simulink model "mcb_hostmodel_dsPIC33A"  (R2025b)
settings: Solver=FixedStepDiscrete  StartTime=0.0  StopTime=inf  RelTol=1e-3  EnableMultiTasking=on
values from neighbouring files (symbols this model uses):
  Ts_serialOut = 500e-6    (= 0.0005)    [mchp_acim_foc_dsPIC33A_data.m]
undefined symbols (not defined in the file or in its folder): target
libraries: instrumentseriallib x3, simulink x3
settings Model: Creator=The MathWorks, Inc.  LastModifiedBy=I73849
settings SolverCC: AlgebraicLoopSolver=TrustRegion  MaxZcPerStep=1.0
settings DataIOCC: LimitDataPoints=on  SaveFormat=Array  ReturnWorkspaceOutputs=off
settings OptimizationCC: ReuseModelBlockBuffer=off  LifeSpan=1  EfficientTunableParamExpr=on
settings DebuggingCC: UnderspecifiedInitializationDetection=Classic  MergeDetectMultiDrivingBlocksExec=none  SolverPrmCheckMsg=warning  ParameterPrecisionLossMsg=none  UnconnectedInputMsg=warning  UnconnectedOutputMsg=warning  UnconnectedLineMsg=warning  AllowSymbolicDim=off  PregeneratedLibrarySubsystemCodeDiagnostic=none  SFUnexpectedBacktrackingDiag=warning  SFNoUnconditionalDefaultTransitionDiag=warning  SFExecutionAtInitializationDiag=none  ArithmeticOperatorsInVariantConditions=warning
settings HardwareCC: ProdBitPerPointer=32.0  ProdLargestAtomicFloat=None  ProdIntDivRoundTo=Undefined  ProdEndianess=Unspecified  ProdWordSize=32.0  ProdHWDeviceType=32-bit Generic
settings ModelReferenceCC: EnableRefExpFcnMdlSchedulingChecks=on  PropagateSignalLabelsOutOfModel=off
settings SFSimCC: SimUseLocalCustomCode=off  MATLABDynamicMemAlloc=off
settings RTWCC: SystemTargetFile=ert.tlc  TemplateMakefile=ert_default_tmf  GenerateReport=on  RTWUseLocalCustomCode=off  IncludeHyperlinkInReport=on  LaunchReport=on  GenerateTraceInfo=on  GenerateTraceReport=on  GenerateTraceReportSl=on  GenerateTraceReportSf=on  GenerateTraceReportEml=on  GPUComputeCapability=3.5  DLArmComputeVersion=19.05  Description=Real-Time Workshop Embedded Coder
settings CodeAppCC: IgnoreCustomStorageClasses=off  StateflowObjectComments=on  InternalIdentifier=Classic
settings ERTTargetCC: InlinedParameterPlacement=Hierarchical  ERTCustomFileTemplate=example_file_process.tlc  ConvertIfToSwitch=off  SuppressUnreachableDefaultCases=off  DynamicArrayContainerType=coder::array  MultiwordLength=2048.0  GenerateSampleERTMain=on
settings ConfigComp: CovMetricSettings=dw  CovSaveCumulativeToWorkspaceVar=on  CovSaveSingleToWorkspaceVar=on  CovExternalEMLEnable=off  CovSFcnEnable=off

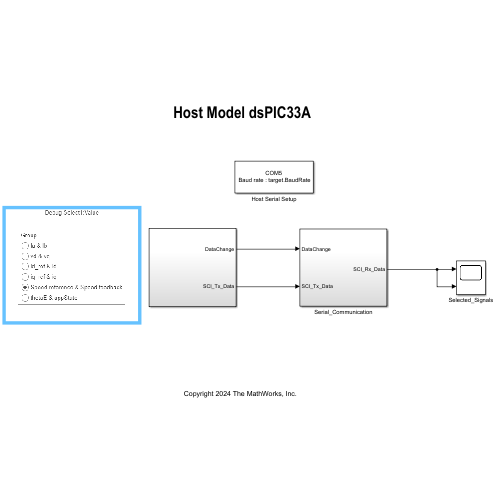
[thumbnail: Simulink's stored preview of the top-level diagram]
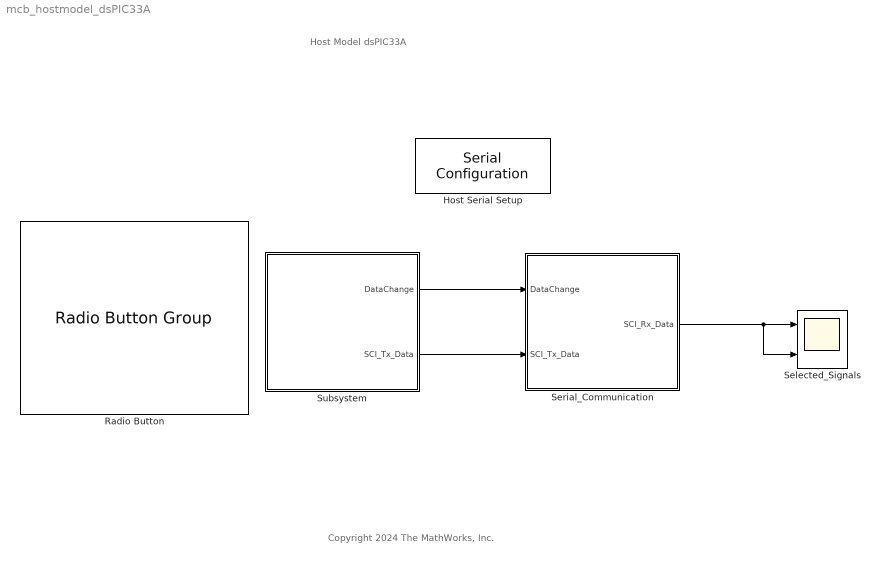
== system mcb_hostmodel_dsPIC33A ==
  note: Host Model dsPIC33A
  note: Copyright 2024 The MathWorks, Inc.
  Host Serial Setup : instrumentseriallib/Serial Configuration  Priority=-99  PortSel=target.comport  Port=target.comport  ComPort=target.comport  BaudRate=target.BaudRate  DataBits=8  Parity=none  StopBits=1  ByteOrder=little-endian  FlowControl=none  Timeout=2  SimulateUsing=Interpreted execution  BlockInModel=on  aMode=5
  Radio Button : RadioButtonGroup  SelectedLabel=Speed reference & Speed feedback  ButtonGroupName=Group
  Selected_Signals : Scope  NumInputPorts=2
      settings: TimeSpan=4  ActiveDisplayYMinimum=-510.99130861461151  ActiveDisplayYMaximum=4605.8121853321791  DataLoggingVariableName=Results_HW
  Serial_Communication : Subsystem
  Subsystem : Subsystem
  wires:
  Subsystem/2(SCI_Tx_Data) -> Serial_Communication/2(SCI_Tx_Data)
  Subsystem/1(DataChange) -> Serial_Communication/1(DataChange)
  Serial_Communication/1(SCI_Rx_Data) -> Selected_Signals/2, Selected_Signals/1

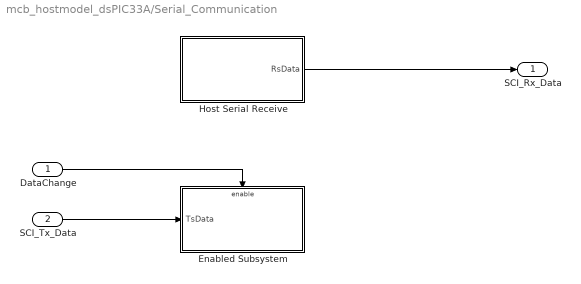
== system mcb_hostmodel_dsPIC33A/Serial_Communication ==
  DataChange : Inport
  SCI_Tx_Data : Inport  Port=2
  Enabled Subsystem : Subsystem  TreatAsAtomicUnit=on
  Host Serial Receive : Subsystem
  SCI_Rx_Data : Outport
  wires:
  DataChange/1 -> Enabled Subsystem/Enable
  SCI_Tx_Data/1 -> Enabled Subsystem/1(TsData)
  Host Serial Receive/1(RsData) -> SCI_Rx_Data/1

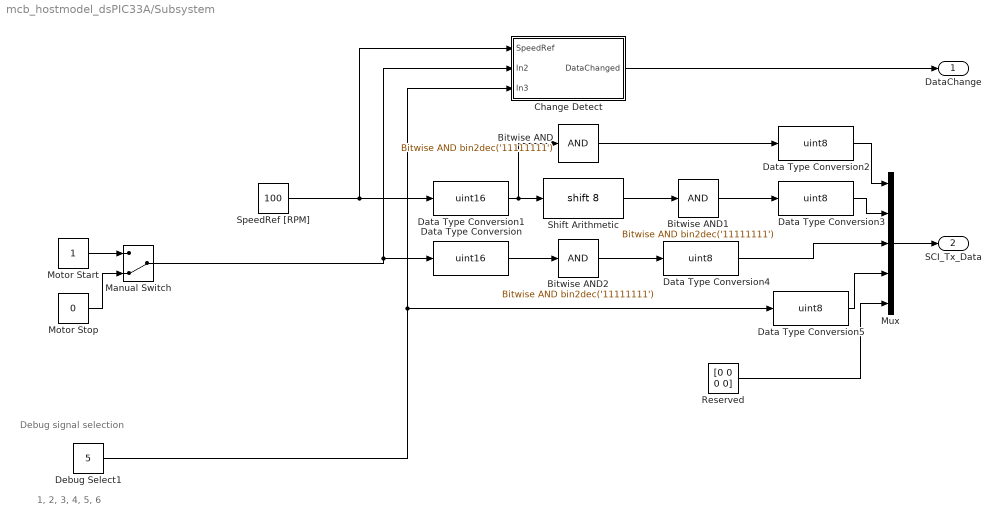
== system mcb_hostmodel_dsPIC33A/Subsystem ==
  note: 1, 2, 3, 4, 5, 6
  note: Debug signal selection
  Bitwise AND : simulink/Logic and Bit Operations/Bitwise Operator  logicop=AND  UseBitMask=on  BitMask=bin2dec('11111111')  BitMaskRealWorld=Stored Integer
  Bitwise AND1 : simulink/Logic and Bit Operations/Bitwise Operator  logicop=AND  UseBitMask=on  BitMask=bin2dec('11111111')  BitMaskRealWorld=Stored Integer
  Bitwise AND2 : simulink/Logic and Bit Operations/Bitwise Operator  logicop=AND  UseBitMask=on  BitMask=bin2dec('11111111')  BitMaskRealWorld=Stored Integer
  Change Detect : Subsystem
  Data Type Conversion : DataTypeConversion  OutDataTypeStr=uint16  ConvertRealWorld=Stored Integer (SI)  RndMeth=Simplest  SaturateOnIntegerOverflow=off
  Data Type Conversion1 : DataTypeConversion  OutDataTypeStr=uint16  ConvertRealWorld=Stored Integer (SI)  RndMeth=Simplest  SaturateOnIntegerOverflow=off
  Data Type Conversion{2..5} (4 alike) : DataTypeConversion  OutDataTypeStr=uint8  ConvertRealWorld=Stored Integer (SI)  RndMeth=Simplest  SaturateOnIntegerOverflow=off
  Debug Select1 : Constant  Value=5  OutDataTypeStr=uint8  SampleTime=-1
  Manual Switch : ManualSwitch  CurrentSetting=0
  Motor Start : Constant  OutDataTypeStr=uint16  SampleTime=-1
  Motor Stop : Constant  Value=0  OutDataTypeStr=uint16  SampleTime=-1
  Mux : Mux  Inputs=5
  Reserved : Constant  Value=[0 0 0 0]  OutDataTypeStr=uint8  SampleTime=-1
  Shift Arithmetic : ArithShift  BitShiftNumber=8
  SpeedRef [RPM] : Constant  Value=100  OutDataTypeStr=int16  SampleTime=-1
  DataChange : Outport
  SCI_Tx_Data : Outport  Port=2
  wires:
  Reserved/1 -> Mux/5
  Data Type Conversion3/1 -> Mux/2
  Data Type Conversion5/1 -> Mux/4
  Data Type Conversion2/1 -> Mux/1
  Debug Select1/1 -> Change Detect/3(In3), Data Type Conversion5/1
  Data Type Conversion4/1 -> Mux/3
  Bitwise AND1/1 -> Data Type Conversion3/1
  Bitwise AND/1 -> Data Type Conversion2/1
  Bitwise AND2/1 -> Data Type Conversion4/1
  Data Type Conversion1/1 -> Bitwise AND/1, Shift Arithmetic/1
  Shift Arithmetic/1 -> Bitwise AND1/1
  Data Type Conversion/1 -> Bitwise AND2/1
  Manual Switch/1 -> Change Detect/2(In2), Data Type Conversion/1
  Mux/1 -> SCI_Tx_Data/1
  Change Detect/1(DataChanged) -> DataChange/1
  SpeedRef [RPM]/1 -> Change Detect/1(SpeedRef), Data Type Conversion1/1
  Motor Start/1 -> Manual Switch/1
  Motor Stop/1 -> Manual Switch/2

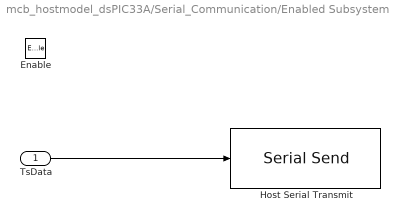
== system mcb_hostmodel_dsPIC33A/Serial_Communication/Enabled Subsystem ==
  TsData : Inport
  Enable : EnablePort
  Host Serial Transmit : instrumentseriallib/Serial Send  PortSel=target.comport  Port=target.comport  ComPort=target.comport  Header=[]  Terminator=<none>  CustomTerminator=[]  EnableBlockingMode=off  SimulateUsing=Interpreted execution  BlockInModel=on  aMode=5
  wires:
  TsData/1 -> Host Serial Transmit/1

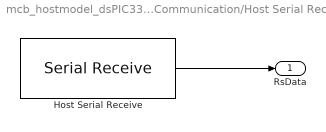
== system mcb_hostmodel_dsPIC33A/Serial_Communication/Host Serial Receive ==
  Host Serial Receive : instrumentseriallib/Serial Receive  PortSel=target.comport  Port=target.comport  ComPort=target.comport  DataType=single  SaveDataType=uint8  ToggleHeader=on  Header='S'  ToggleDataSize=on  DataSize=[target.frameSize 2]  ToggleTerminator=on  Terminator=Custom terminator  CustomTerminator='E'  InputFormat=Row major  EnableBlockingMode=on  ActionDataUnavailable=Output custom value  ActionWhenDataUnavailable=Output custom value  CustomValue=4  SampleTime=target.frameSize * Ts_serialOut  SimulateUsing=Interpreted execution  BlockInModel=on  aMode=5  LibraryInUse=instrumentlib
  RsData : Outport
  wires:
  Host Serial Receive/1 -> RsData/1

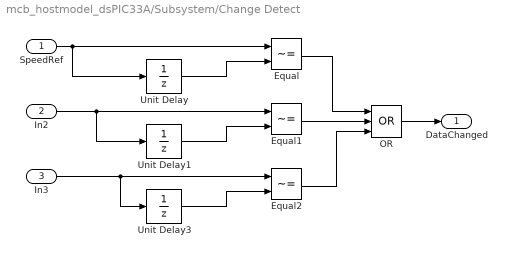
== system mcb_hostmodel_dsPIC33A/Subsystem/Change Detect ==
  SpeedRef : Inport
  In2 : Inport  Port=2
  In3 : Inport  Port=3
  Equal : RelationalOperator  Operator=~=  OutDataTypeStr=boolean  RndMeth=Simplest  InputSameDT=off
  Equal1 : RelationalOperator  Operator=~=  OutDataTypeStr=boolean  RndMeth=Simplest  InputSameDT=off
  Equal2 : RelationalOperator  Operator=~=  OutDataTypeStr=boolean  RndMeth=Simplest  InputSameDT=off
  OR : Logic  Operator=OR  Inputs=3  IconShape=distinctive  AllPortsSameDT=off  OutDataTypeStr=boolean
  Unit Delay : UnitDelay  SampleTime=-1  HasFrameUpgradeWarning=on
  Unit Delay1 : UnitDelay  SampleTime=-1  HasFrameUpgradeWarning=on
  Unit Delay3 : UnitDelay  SampleTime=-1  HasFrameUpgradeWarning=on
  DataChanged : Outport
  wires:
  Equal2/1 -> OR/3
  OR/1 -> DataChanged/1
  In3/1 -> Unit Delay3/1, Equal2/1
  Equal1/1 -> OR/2
  Unit Delay/1 -> Equal/2
  Equal/1 -> OR/1
  In2/1 -> Unit Delay1/1, Equal1/1
  SpeedRef/1 -> Unit Delay/1, Equal/1
  Unit Delay1/1 -> Equal1/2
  Unit Delay3/1 -> Equal2/2
